simulink model "uav_6dof_course"  (R2024a)
settings: Solver=FixedStepDiscrete  StartTime=0  StopTime=20  FixedStep=0.01  RelTol=1e-3
settings Model: Creator=32686  LastModifiedBy=32686

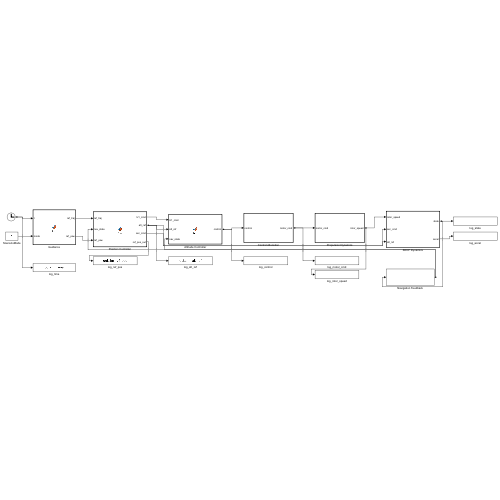
[thumbnail: Simulink's stored preview of the top-level diagram]
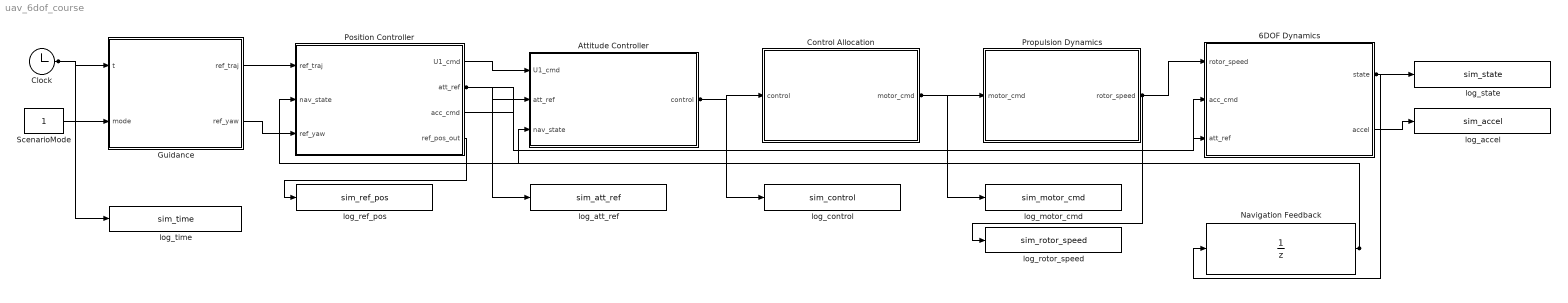
== system uav_6dof_course ==
  6DOF Dynamics : MATLAB Function  TreatAsAtomicUnit=on
  Attitude Controller : MATLAB Function  TreatAsAtomicUnit=on
  Clock : Clock
  Control Allocation : MATLAB Function  TreatAsAtomicUnit=on
  Guidance : MATLAB Function  TreatAsAtomicUnit=on
  Navigation Feedback : UnitDelay  InitialCondition=[0;0;0;0;0;0;0;0;0;0;0;0]  SampleTime=0.01  HasFrameUpgradeWarning=on
  Position Controller : MATLAB Function  TreatAsAtomicUnit=on
  Propulsion Dynamics : MATLAB Function  TreatAsAtomicUnit=on
  ScenarioMode : Constant
  log_accel : ToWorkspace  VariableName=sim_accel  SaveFormat=Timeseries  SampleTime=-1
  log_att_ref : ToWorkspace  VariableName=sim_att_ref  SaveFormat=Timeseries  SampleTime=-1
  log_control : ToWorkspace  VariableName=sim_control  SaveFormat=Timeseries  SampleTime=-1
  log_motor_cmd : ToWorkspace  VariableName=sim_motor_cmd  SaveFormat=Timeseries  SampleTime=-1
  log_ref_pos : ToWorkspace  VariableName=sim_ref_pos  SaveFormat=Timeseries  SampleTime=-1
  log_rotor_speed : ToWorkspace  VariableName=sim_rotor_speed  SaveFormat=Timeseries  SampleTime=-1
  log_state : ToWorkspace  VariableName=sim_state  SaveFormat=Timeseries  SampleTime=-1
  log_time : ToWorkspace  VariableName=sim_time  SaveFormat=Timeseries  SampleTime=-1
  wires:
  Clock/1 -> Guidance/1(t), log_time/1
  ScenarioMode/1 -> Guidance/2(mode)
  Guidance/1(ref_traj) -> Position Controller/1(ref_traj)
  Guidance/2(ref_yaw) -> Position Controller/3(ref_yaw)
  Navigation Feedback/1 -> Position Controller/2(nav_state), Attitude Controller/3(nav_state)
  Position Controller/1(U1_cmd) -> Attitude Controller/1(U1_cmd)
  Position Controller/2(att_ref) -> Attitude Controller/2(att_ref), 6DOF Dynamics/3(att_ref), log_att_ref/1
  Attitude Controller/1(control) -> Control Allocation/1(control), log_control/1
  Control Allocation/1(motor_cmd) -> Propulsion Dynamics/1(motor_cmd), log_motor_cmd/1
  Propulsion Dynamics/1(rotor_speed) -> 6DOF Dynamics/1(rotor_speed), log_rotor_speed/1
  Position Controller/3(acc_cmd) -> 6DOF Dynamics/2(acc_cmd)
  6DOF Dynamics/1(state) -> Navigation Feedback/1, log_state/1
  Position Controller/4(ref_pos_out) -> log_ref_pos/1
  6DOF Dynamics/2(accel) -> log_accel/1

== matlab function uav_6dof_course/Position Controller ==
  data: ref_traj input; U1_cmd output; nav_state input; ref_yaw input; att_ref output; acc_cmd output; ref_pos_out output
function [U1_cmd, att_ref, acc_cmd, ref_pos_out] = fcn(ref_traj, nav_state, ref_yaw)
m = 1.2; g = 9.8; dt = 0.01;
persistent integ_pos
if isempty(integ_pos)
    integ_pos = zeros(3,1);
end
pos = nav_state(1:3); vel = nav_state(4:6);
ref_pos = ref_traj(1:3); ref_vel = ref_traj(4:6); ref_acc = ref_traj(7:9);
kp = [0.55; 0.55; 1.80]; ki = [0.00; 0.00; 0.01]; kd = [1.65; 1.65; 2.35];
err = ref_pos - pos;
integ_pos = min(max(integ_pos + err*dt, -2), 2);
vel_err = ref_vel - vel;
acc_cmd = ref_acc + kp.*err + ki.*integ_pos + kd.*vel_err;
acc_cmd(1) = min(max(acc_cmd(1), -0.80), 0.80);
acc_cmd(2) = min(max(acc_cmd(2), -0.80), 0.80);
acc_cmd(3) = min(max(acc_cmd(3), -4.0), 4.0);
yaw = ref_yaw;
phi_ref = (acc_cmd(1)*sin(yaw) - acc_cmd(2)*cos(yaw))/g;
theta_ref = (acc_cmd(1)*cos(yaw) + acc_cmd(2)*sin(yaw))/g;
phi_ref = min(max(phi_ref, -0.12), 0.12);
theta_ref = min(max(theta_ref, -0.12), 0.12);
att_ref = [phi_ref; theta_ref; yaw];
U1_cmd = min(max(m*(g + acc_cmd(3)), 0.2*m*g), 1.8*m*g);
ref_pos_out = ref_pos;
end

== matlab function uav_6dof_course/Guidance ==
  data: t input; ref_traj output; mode input; ref_yaw output
function [ref_traj, ref_yaw] = fcn(t, mode)
% ref_traj = [position; velocity; acceleration].
ref_yaw = 0;
x = 0; y = 0; z = 3; vx = 0; vy = 0; vz = 0; ax = 0; ay = 0; az = 0;
if mode < 1.5
    [z, vz, az] = quintic_segment(t, 0, 5, 0, 3);
elseif mode < 2.5
    [z, vz, az] = quintic_segment(t, 0, 5, 0, 3);
    [x, vx, ax] = quintic_segment(t, 5, 18, 0, 6);
elseif mode < 3.5
    [z, vz, az] = quintic_segment(t, 0, 5, 0, 3);
    [z2, vz2, az2] = quintic_segment(t, 8, 16, 3, 5);
    if t >= 8
        z = z2; vz = vz2; az = az2;
    end
else
    [z, vz, az] = quintic_segment(t, 0, 5, 0, 3);
    [y, vy, ay] = quintic_segment(t, 5, 17, 0, 3);
end
ref_traj = [x; y; z; vx; vy; vz; ax; ay; az];
end

function [p, v, a] = quintic_segment(t, t0, tf, p0, pf)
if t <= t0
    p = p0; v = 0; a = 0;
elseif t >= tf
    p = pf; v = 0; a = 0;
else
    T = tf - t0;
    s = (t - t0) / T;
    ds = 1 / T;
    h = 10*s^3 - 15*s^4 + 6*s^5;
    hd = (30*s^2 - 60*s^3 + 30*s^4) * ds;
    hdd = (60*s - 180*s^2 + 120*s^3) * ds * ds;
    p = p0 + (pf - p0) * h;
    v = (pf - p0) * hd;
    a = (pf - p0) * hdd;
end
end

== matlab function uav_6dof_course/Attitude Controller ==
  data: U1_cmd input; control output; att_ref input; nav_state input
function control = fcn(U1_cmd, att_ref, nav_state)
control = zeros(4,1);
dt = 0.01;
persistent integ_att
if isempty(integ_att)
    integ_att = zeros(3,1);
end
eul = nav_state(7:9); omega = nav_state(10:12);
kp = [6.2; 6.2; 3.2]; ki = [0.0; 0.0; 0.0]; kd = [2.8; 2.8; 1.6];
err = att_ref - eul;
err(3) = atan2(sin(err(3)), cos(err(3)));
integ_att = min(max(integ_att + err*dt, -1), 1);
tau = kp.*err + ki.*integ_att - kd.*omega;
tau = min(max(tau, [-0.8; -0.8; -0.25]), [0.8; 0.8; 0.25]);
control(:) = [U1_cmd; tau];
end

== matlab function uav_6dof_course/Control Allocation ==
  data: control input; motor_cmd output
function motor_cmd = fcn(control)
motor_cmd = zeros(4,1);
kf = 3.1e-5; l = 0.25; km = 1.2e-6;
U1 = control(1); tau = control(2:4);
w2cmd = zeros(4,1);
w2cmd(1) = U1/(4*kf) - tau(2)/(2*kf*l) + tau(3)/(4*km);
w2cmd(2) = U1/(4*kf) + tau(1)/(2*kf*l) - tau(3)/(4*km);
w2cmd(3) = U1/(4*kf) + tau(2)/(2*kf*l) + tau(3)/(4*km);
w2cmd(4) = U1/(4*kf) - tau(1)/(2*kf*l) - tau(3)/(4*km);
w2cmd = min(max(w2cmd, 0), 900^2);
motor_cmd(:) = sqrt(w2cmd);
end

== matlab function uav_6dof_course/Propulsion Dynamics ==
  data: motor_cmd input; rotor_speed output
function rotor_speed = fcn(motor_cmd)
rotor_speed = zeros(4,1);
persistent w
dt = 0.01; tau = 0.10;
if isempty(w)
    w = zeros(4,1);
end
w = w + dt/tau*(motor_cmd - w);
rotor_speed(:) = w;
end

== matlab function uav_6dof_course/6DOF Dynamics ==
  data: rotor_speed input; state output; acc_cmd input; att_ref input; accel output
function [state, accel] = fcn(rotor_speed, acc_cmd, att_ref)
% 6DOF rigid-body dynamics driven by rotor thrust and torque.
% acc_cmd and att_ref are retained for the subsystem interface/logging chain.
persistent x
dt = 0.01; m = 1.2; g = 9.8;
kf = 3.1e-5; l = 0.25; km = 1.2e-6;
I = [0.025; 0.025; 0.045];
lin_drag = [0.10; 0.10; 0.16]; ang_drag = [0.015; 0.015; 0.020];
if isempty(x)
    x = zeros(12,1);
end
pos = x(1:3); vel = x(4:6); eul = x(7:9); omega = x(10:12);
phi = eul(1); theta = eul(2); psi = eul(3);
w2 = rotor_speed(:).*rotor_speed(:);
f = kf*w2;
U1 = sum(f);
tau = [l*kf*(w2(2)-w2(4)); l*kf*(w2(3)-w2(1)); km*(w2(1)-w2(2)+w2(3)-w2(4))];
cphi = cos(phi); sphi = sin(phi); cth = cos(theta); sth = sin(theta); cpsi = cos(psi); spsi = sin(psi);
R = [cpsi*cth, cpsi*sth*sphi-spsi*cphi, cpsi*sth*cphi+spsi*sphi;
     spsi*cth, spsi*sth*sphi+cpsi*cphi, spsi*sth*cphi-cpsi*sphi;
     -sth,     cth*sphi,                    cth*cphi];
thrust_inertial = R*[0;0;U1];
acc = thrust_inertial/m - [0;0;g] - lin_drag.*vel;
gyro = cross(omega, I.*omega);
omega_dot = (tau - gyro - ang_drag.*omega)./I;
cth_safe = sign(cth)*max(abs(cth), 0.05);
eul_dot = [1, sphi*tan(theta), cphi*tan(theta);
           0, cphi,           -sphi;
           0, sphi/cth_safe,   cphi/cth_safe] * omega;
vel = vel + acc*dt;
pos = pos + vel*dt;
omega = omega + omega_dot*dt;
eul = eul + eul_dot*dt;
eul(3) = atan2(sin(eul(3)), cos(eul(3)));
x = [pos; vel; eul; omega];
state = x;
accel = [acc; omega_dot];
end
